simulink model "simulink_app"  (R2015a)
settings: Solver=FixedStepDiscrete  SolverMode=SingleTasking  StartTime=0.0  StopTime=inf  FixedStep=0.004  RelTol=1e-3
undefined symbols (not defined in the file): T_ctrl
libraries: simulink x6
settings Model: Creator=Adam  LastModifiedBy=David
settings SolverCC: AutoInsertRateTranBlk=on
settings DataIOCC: LimitDataPoints=off  SignalLoggingSaveFormat=ModelDataLogs  SaveOutput=off  SignalLogging=off  DSMLogging=off  SaveTime=off
settings OptimizationCC: InlineParams=on  OptimizeModelRefInitCode=on  LifeSpan=Inf
settings DebuggingCC: UnderspecifiedInitializationDetection=Classic  MergeDetectMultiDrivingBlocksExec=none  SolverPrmCheckMsg=warning  MultiTaskDSMMsg=warning  MultiTaskCondExecSysMsg=none  UnconnectedInputMsg=none  UnconnectedOutputMsg=none  UnconnectedLineMsg=none  StateNameClashWarn=warning  StrictBusMsg=None
settings HardwareCC: ProdLargestAtomicInteger=Long  ProdLargestAtomicFloat=Float  ProdEndianess=LittleEndian  ProdHWDeviceType=ARM Compatible->ARM 7
settings RTWCC: SystemTargetFile=ert.tlc  GenCodeOnly=on  GenerateMakefile=off  TemplateMakefile=ert_default_tmf  Description=Embedded Coder  RTWVerbose=off  RTWCompilerOptimization=on
settings RTWCC: CustomSourceCode=|
  | // Simulink wrapper code for PX4 (PX4FMU & Pixhawk)
  | // Developed by Adam Polak, Polakium Engineering 2014
  | // http://www.polakiumengineering.org
  | 
  | #include <nuttx/config.h>
  | #include <poll.h>
  | #include <stdio.h>
  | #include <stdlib.h>
  | #include <unistd.h>
  | #include <uORB/uORB.h>
  | #include <uORB/topics/sensor_combined.h>
  | #include <uORB/topics/vehicle_attitude.h>
  | #include <uORB/topics/optical_flow.h>
  | #include <uORB/topics/vehicle_gps_position.h>
  | #include <drivers/drv_led.h>
  | #include <drivers/drv_rgbled.h>
  | #include <drivers/drv_pwm_output.h>
  | #include <drivers/drv_rc_input.h>
  | #include <drivers/drv_hrt.h>
  | #include <systemlib/systemlib.h>
  | 
  | __EXPORT int simulink_app_main(int argc, char *argv[]);
  | 
  | const char *dev_rgbled = RGBLED_DEVICE_PATH;
  | const char *dev_pwm = PWM_OUTPUT_DEVICE_PATH;
  | 
  | static int simulink_task;
  | static bool thread_exit;
  | static bool pwm_enabled;
  | 
  | struct rgbled_rgbset_t{
  |   uint8_t red;
  |   uint8_t green;
  |   uint8_t blue;
  | };
  | 
  | int step_size = 4; // fundamental sample time (ms)
  | int i = 1;
  | 
  | int simulink_main(int argc, char *argv[])
  | {
  |   simulink_app_initialize();
  | 
  |   // declare data subscriptions
  |   int sensors_sub = orb_subscribe(ORB_ID(sensor_combined));
  |   int pwm_inputs_sub = orb_subscribe(ORB_ID(input_rc));
  |   int attitude_sub = orb_subscribe(ORB_ID(vehicle_attitude));
  |   int flow_sub = orb_subscribe(ORB_ID(optical_flow));
  |   int gps_sub = orb_subscribe(ORB_ID(vehicle_gps_position));
  | 
  |   struct sensor_combined_s sensors;
  |   struct rc_input_values pwm_inputs;
  |   struct vehicle_attitude_s attitude;
  |   struct optical_flow_s flow;
  |   struct vehicle_gps_position_s gps;
  | 
  |   orb_set_interval(sensors_sub, step_size);
  | 
  |   // declare output devices
  |   int rgbled = open(dev_rgbled, 0);
  |   int pwm = open(dev_pwm, 0);
  | 
  |   // initialize outputs
  |   ioctl(rgbled, RGBLED_SET_MODE, (unsigned long)RGBLED_MODE_ON);
  |   ioctl(pwm, PWM_SERVO_SET_ARM_OK, 0);
  |   ioctl(pwm, PWM_SERVO_ARM, 0);
  |   pwm_enabled = 0;
  | 
  |   struct pollfd fds[] = {
  |     { .fd = sensors_sub, .events = POLLIN },
  |   };
  | 
  |   // primary application thread
  |   while (!thread_exit) {
  |     int poll_return = poll(fds, 1, 1000);
  |     if (poll_return > 0) {
  |       if (fds[0].revents & POLLIN) {
  |         // assign sensor data
  |         orb_copy(ORB_ID(sensor_combined), sensors_sub, &sensors);
  |         orb_copy(ORB_ID(vehicle_attitude), attitude_sub, &attitude);
  |         orb_copy(ORB_ID(optical_flow), flow_sub, &flow);
  |         orb_copy(ORB_ID(vehicle_gps_position), gps_sub, &gps);
  |         orb_copy(ORB_ID(input_rc), pwm_inputs_sub, &pwm_inputs);
  |         simulink_app_U.runtime = hrt_absolute_time();
  |         simulink_app_U.mag_x = sensors.magnetometer_ga[0];
  |         simulink_app_U.mag_y = sensors.magnetometer_ga[1];
  |         simulink_app_U.mag_z = sensors.magnetometer_ga[2];
  |         simulink_app_U.acc_x = sensors.accelerometer_m_s2[0];
  |         simulink_app_U.acc_y = sensors.accelerometer_m_s2[1];
  |         simulink_app_U.acc_z = sensors.accelerometer_m_s2[2];
  |         simulink_app_U.gyro_x = sensors.gyro_rad_s[0];
  |         simulink_app_U.gyro_y = sensors.gyro_rad_s[1];
  |         simulink_app_U.gyro_z = sensors.gyro_rad_s[2];
  |         simulink_app_U.rate_roll = attitude.rollspeed;
  |         simulink_app_U.rate_pitch = attitude.pitchspeed;
  |         simulink_app_U.rate_yaw = attitude.yawspeed;
  |         simulink_app_U.att_roll = attitude.roll;
  |         simulink_app_U.att_pitch = attitude.pitch;
  |         simulink_app_U.att_yaw = attitude.yaw;
  |         simulink_app_U.q0 = attitude.q[0];
  |         simulink_app_U.q1 = attitude.q[1];
  |         simulink_app_U.q2 = attitude.q[2];
  |         simulink_app_U.q3 = attitude.q[3];
  |         simulink_app_U.baro_alt = sensors.baro_alt_meter;
  |         simulink_app_U.sonar_dist = flow.ground_distance_m;
  |         simulink_app_U.flow_x = flow.flow_comp_x_m;
  |         simulink_app_U.flow_y = flow.flow_comp_y_m;
  |         simulink_app_U.gps_sat = gps.satellites_used;
  |         simulink_app_U.gps_lat = 0.0000001*(double)gps.lat;
  |         simulink_app_U.gps_lon = 0.0000001*(double)gps.lon;
  |         simulink_app_U.gps_alt = 0.001*(double)gps.alt;
  |         simulink_app_U.gps_vel = gps.vel_m_s;
  |         simulink_app_U.gps_vel_n = gps.vel_n_m_s;
  |         simulink_app_U.gps_vel_e = gps.vel_e_m_s;
  |         simulink_app_U.gps_vel_d = gps.vel_d_m_s;
  |         simulink_app_U.ch1 = pwm_inputs.values[0];
  |         simulink_app_U.ch2 = pwm_inputs.values[1];
  |         simulink_app_U.ch3 = pwm_inputs.values[2];
  |         simulink_app_U.ch4 = pwm_inputs.values[3];
  |         simulink_app_U.ch5 = pwm_inputs.values[4];
  |         simulink_app_U.ch6 = pwm_inputs.values[5];
  |         simulink_app_U.ch7 = pwm_inputs.values[6];
  |         simulink_app_U.ch8 = pwm_inputs.values[7];
  |         if (i < 25) { // 10Hz loop
  |           i = i++;
  |         } else {
  |           // check arm state
  |           if (simulink_app_Y.pwm_arm == 1 && pwm_enabled == 0) {
  |             // arm system
  |             pwm_enabled = 1;
  |             printf("\t  ARMED\t\t  ARMED\t\t  ARMED\t\t  ARMED\t\t  ARMED\t\t  ARMED\t\t  ARMED\t\t  ARMED\n");
  |           } else if (simulink_app_Y.pwm_arm == 0 && pwm_enabled == 1) {
  |             // disarm system
  |             ioctl(pwm, PWM_SERVO_SET(0), 1000);
  |             ioctl(pwm, PWM_SERVO_SET(1), 1000);
  |             ioctl(pwm, PWM_SERVO_SET(2), 1000);
  |             ioctl(pwm, PWM_SERVO_SET(3), 1000);
  |             ioctl(pwm, PWM_SERVO_SET(4), 1000);
  |             ioctl(pwm, PWM_SERVO_SET(5), 1000);
  |             ioctl(pwm, PWM_SERVO_SET(6), 1000);
  |             ioctl(pwm, PWM_SERVO_SET(7), 1000);
  |             pwm_enabled = 0;
  |             printf("\tDISARMED\tDISARMED\tDISARMED\tDISARMED\tDISARMED\tDISARMED\tDISARMED\tDISARMED\n");
  |           }
  |           // output FMU LED signals
  |           if (simulink_app_Y.led_blue == 1) {
  |             led_on(LED_BLUE);
  |           } else {
  |             led_off(LED_BLUE);
  |           }
  |           if (simulink_app_Y.led_red == 1) {
  |             led_on(LED_RED);
  |           } else {
  |             led_off(LED_RED);
  |           }
  |           // output RGBLED signals
  |           rgbled_rgbset_t rgb_value;
  |           rgb_value.red = simulink_app_Y.rgb_red;
  |           rgb_value.green = simulink_app_Y.rgb_green;
  |           rgb_value.blue = simulink_app_Y.rgb_blue;
  |           ioctl(rgbled, RGBLED_SET_RGB, (unsigned long)&rgb_value);
  |           //print debug data
  |           printf("%8.4f\t%8.4f\t%8.4f\t%8.4f\t%8.4f\t%8.4f\t%8.4f\t%8.4f\t%8.4f\n",
  |               (double)(simulink_app_U.runtime/1000000),
  |               (double)simulink_app_Y.debug1,
  |               (double)simulink_app_Y.debug2,
  |               (double)simulink_app_Y.debug3,
  |               (double)simulink_app_Y.debug4,
  |               (double)simulink_app_Y.debug5,
  |               (double)simulink_app_Y.debug6,
  |               (double)simulink_app_Y.debug7,
  |               (double)simulink_app_Y.debug8);
  |           i = 1;
  |         }
  |         // output pwm signals
  |         if (pwm_enabled == 1) {
  |           ioctl(pwm, PWM_SERVO_SET(0), simulink_app_Y.pwm1);
  |           ioctl(pwm, PWM_SERVO_SET(1), simulink_app_Y.pwm2);
  |           ioctl(pwm, PWM_SERVO_SET(2), simulink_app_Y.pwm3);
  |           ioctl(pwm, PWM_SERVO_SET(3), simulink_app_Y.pwm4);
  |           ioctl(pwm, PWM_SERVO_SET(4), simulink_app_Y.pwm5);
  |           ioctl(pwm, PWM_SERVO_SET(5), simulink_app_Y.pwm6);
  |           ioctl(pwm, PWM_SERVO_SET(6), simulink_app_Y.pwm7);
  |           ioctl(pwm, PWM_SERVO_SET(7), simulink_app_Y.pwm8);
  |         } else {
  |           ioctl(pwm, PWM_SERVO_SET(0), 1000);
  |           ioctl(pwm, PWM_SERVO_SET(1), 1000);
  |           ioctl(pwm, PWM_SERVO_SET(2), 1000);
  |           ioctl(pwm, PWM_SERVO_SET(3), 1000);
  |           ioctl(pwm, PWM_SERVO_SET(4), 1000);
  |           ioctl(pwm, PWM_SERVO_SET(5), 1000);
  |           ioctl(pwm, PWM_SERVO_SET(6), 1000);
  |           ioctl(pwm, PWM_SERVO_SET(7), 1000);
  |         }
  |         // execute simulink code
  |         simulink_app_step();
  |       }
  |     }
  |   }
  |   // disable pwm outputs
  |   ioctl(pwm, PWM_SERVO_SET(0), 1000);
  |   ioctl(pwm, PWM_SERVO_SET(1), 1000);
  |   ioctl(pwm, PWM_SERVO_SET(2), 1000);
  |   ioctl(pwm, PWM_SERVO_SET(3), 1000);
  |   ioctl(pwm, PWM_SERVO_SET(4), 1000);
  |   ioctl(pwm, PWM_SERVO_SET(5), 1000);
  |   ioctl(pwm, PWM_SERVO_SET(6), 1000);
  |   ioctl(pwm, PWM_SERVO_SET(7), 1000);
  |   ioctl(pwm, PWM_SERVO_DISARM, 0);
  |   // disable LEDs
  |   led_off(LED_BLUE);
  |   led_off(LED_RED);
  |   ioctl(rgbled, RGBLED_SET_MODE, (unsigned long)RGBLED_MODE_OFF);
  |   // close sensor subscriptions
  |   close(sensors_sub);
  |   close(attitude_sub);
  |   close(flow_sub);
  |   close(pwm_inputs_sub);
  |   close(gps_sub);
  |   // terminate application thread
  |   exit(0);
  | }
  | 
  | int simulink_app_main(int argc, char *argv[])
  | {
  |   // start primary application thread
  |   if (!strcmp(argv[1], "start")) {
  |     thread_exit = false;
  |     simulink_task = task_spawn_cmd("simulink_app",
  |       SCHED_DEFAULT,
  |       SCHED_PRIORITY_MAX - 15,
  |       10240,
  |       simulink_main,
  |       NULL);
  |     exit(0);
  |   }
  | 
  |   // terminate primary application thread
  |   if (!strcmp(argv[1], "stop")) {
  |     thread_exit = true;
  |     exit(0);
  |   }
  | 
  |   exit(1);
  | }
settings CodeAppCC: IgnoreCustomStorageClasses=off  SimulinkBlockComments=off
settings ERTTargetCC: GenerateSampleERTMain=off  ParMdlRefBuildCompliant=on  CompOptLevelCompliant=on  ConcurrentExecutionCompliant=on  ERTFirstTimeCompliant=on  SupportContinuousTime=off  SupportVariableSizeSignals=off  ParenthesesLevel=Minimum  ModelStepFunctionPrototypeControlCompliant=on  CPPClassGenCompliant=on  InlinedParameterPlacement=Hierarchical  ERTCustomFileTemplate=example_file_process.tlc  GlobalDataDefinition=InSourceFile  GlobalDataReference=InSourceFile  ERTFilePackagingFormat=Compact  PreserveExternInFcnDecls=off

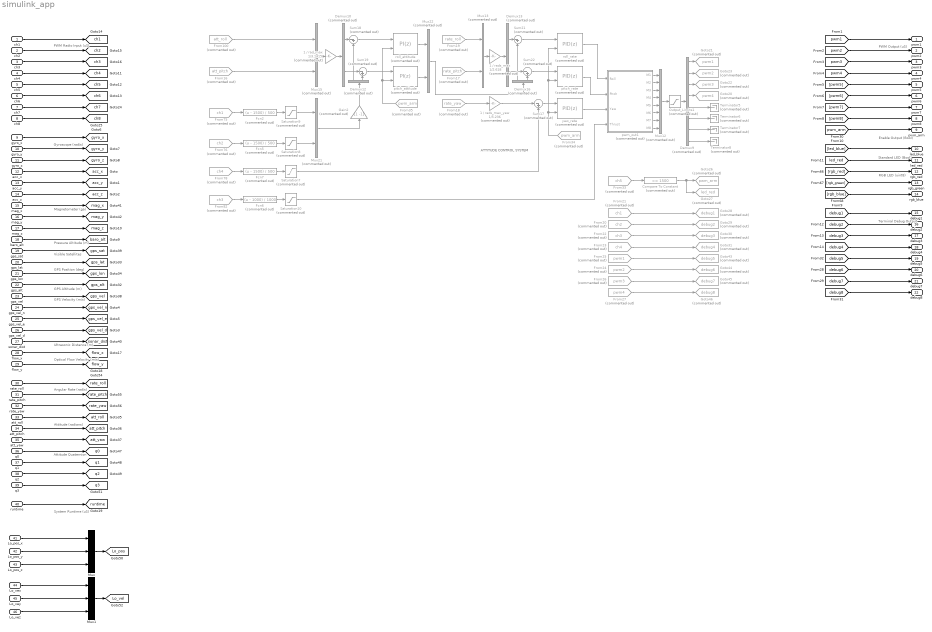
== system simulink_app ==
  note: Terminal Debug Output
  note: RGB LED (uint8)
  note: Standard LED (Bool)
  note: PWM Output (uS)
  note: Enable Output (Bool)
  note: GPS Velocity (m/s)
  note: GPS Altitude (m)
  note: GPS Position (deg)
  note: Attitude Quaternion
  note: Attitude (radians)
  note: Angular Rate (rad/s)
  note: Optical Flow Velocity (m/s)
  note: Ultrasonic Distance (m)
  note: Pressure Altitude (m)
  note: Magnetometer (ga)
  note: System Runtime (uS)
  note: Gyroscope (rad/s)
  note: PWM Radio Input (uS)
  note: Visible Satellites
  note: ATTITUDE CONTROL SYSTEM
  ch1 : Inport
  ch2 : Inport  Port=2
  ch3 : Inport  Port=3
  ch4 : Inport  Port=4
  ch5 : Inport  Port=5
  ch6 : Inport  Port=6
  ch7 : Inport  Port=7
  ch8 : Inport  Port=8
  gyro_x : Inport  Port=9
  gyro_y : Inport  Port=10
  gyro_z : Inport  Port=11
  acc_x : Inport  Port=12
  acc_y : Inport  Port=13
  acc_z : Inport  Port=14
  mag_x : Inport  Port=15
  mag_y : Inport  Port=16
  mag_z : Inport  Port=17
  baro_alt : Inport  Port=18
  gps_sat : Inport  Port=19
  gps_lat : Inport  Port=20
  gps_lon : Inport  Port=21
  gps_alt : Inport  Port=22
  gps_vel : Inport  Port=23
  gps_vel_n : Inport  Port=24
  gps_vel_e : Inport  Port=25
  gps_vel_d : Inport  Port=26
  sonar_dist : Inport  Port=27
  flow_x : Inport  Port=28
  flow_y : Inport  Port=29
  rate_roll : Inport  Port=30
  rate_pitch : Inport  Port=31
  rate_yaw : Inport  Port=32
  att_roll : Inport  Port=33
  att_pitch : Inport  Port=34
  att_yaw : Inport  Port=35
  q0 : Inport  Port=36
  q1 : Inport  Port=37
  q2 : Inport  Port=38
  q3 : Inport  Port=39
  runtime : Inport  Port=40
  Lo_pos_x : Inport  Port=41  PortDimensions=[1,1]  SampleTime=T_ctrl
  Lo_pos_y : Inport  Port=42  PortDimensions=[1,1]  SampleTime=T_ctrl
  Lo_pos_z : Inport  Port=43  PortDimensions=[1,1]  SampleTime=T_ctrl
  Lo_vex : Inport  Port=44  PortDimensions=[1,1]  SampleTime=T_ctrl
  Lo_vey : Inport  Port=45  PortDimensions=[1,1]  SampleTime=T_ctrl
  Lo_vez : Inport  Port=46  PortDimensions=[1,1]  SampleTime=T_ctrl
  1 / rad_max : Gain  Commented=on  Gain=1/3.1415
  1 / rads_max : Gain  Commented=on  Gain=1/2.618
  1 / rads_max_yaw : Gain  Commented=on  Gain=1/5.236
  Compare To Constant : simulink/Logic and Bit Operations/Compare To Constant  Commented=on  relop=>=  const=1500  OutDataTypeStr=boolean
  Demux{10,12..13,16} (4 alike) : Demux  Commented=on  Outputs=2
  Demux9 : Demux  Commented=on  Outputs=8
  Fcn2 : Fcn  Commented=on  Expr=(u - 1500) / 500
  Fcn5 : Fcn  Commented=on  Expr=(u - 1500) / 500
  Fcn6 : Fcn  Commented=on  Expr=(u - 1000) / 1000
  Fcn7 : Fcn  Commented=on  Expr=(u - 1500) / 500
  From100 : From  Commented=on  GotoTag=att_roll  TagVisibility=global
  From16 : From  Commented=on  GotoTag=att_pitch  TagVisibility=global
  From17 : From  Commented=on  GotoTag=rate_pitch  TagVisibility=global
  From18 : From  Commented=on  GotoTag=rate_yaw  TagVisibility=global
  From19 : From  Commented=on  GotoTag=rate_roll  TagVisibility=global
  From20 : From  Commented=on  GotoTag=ch2  TagVisibility=global
  From21 : From  Commented=on  GotoTag=ch1  TagVisibility=global
  From22 : From  Commented=on  GotoTag=ch3  TagVisibility=global
  From23 : From  Commented=on  GotoTag=ch4  TagVisibility=global
  From24 : From  Commented=on  GotoTag=pwm2  TagVisibility=global
  From25 : From  Commented=on  GotoTag=pwm1  TagVisibility=global
  From26 : From  Commented=on  GotoTag=pwm3  TagVisibility=global
  From27 : From  Commented=on  GotoTag=pwm4  TagVisibility=global
  From33 : From  Commented=on  GotoTag=ch5  TagVisibility=global
  From34 : From  Commented=on  GotoTag=pwm_arm  TagVisibility=global
  From35 : From  Commented=on  GotoTag=pwm_arm  TagVisibility=global
  From75 : From  Commented=on  GotoTag=ch1  TagVisibility=global
  From76 : From  Commented=on  GotoTag=ch2  TagVisibility=global
  From78 : From  Commented=on  GotoTag=ch4  TagVisibility=global
  From82 : From  Commented=on  GotoTag=ch3  TagVisibility=global
  Gain2 : Gain  Commented=on  Gain=[1 -1]
  Goto20 : Goto  Commented=on  GotoTag=pwm4  TagVisibility=global
  Goto21 : Goto  Commented=on  GotoTag=pwm1  TagVisibility=global
  Goto22 : Goto  Commented=on  GotoTag=pwm3  TagVisibility=global
  Goto23 : Goto  Commented=on  GotoTag=pwm2  TagVisibility=global
  Goto26 : Goto  Commented=on  GotoTag=pwm_arm  TagVisibility=global
  Goto27 : Goto  Commented=on  GotoTag=led_red  TagVisibility=global
  Goto28 : Goto  Commented=on  GotoTag=debug1  TagVisibility=global
  Goto29 : Goto  Commented=on  GotoTag=debug2  TagVisibility=global
  Goto30 : Goto  Commented=on  GotoTag=debug3  TagVisibility=global
  Goto31 : Goto  Commented=on  GotoTag=debug4  TagVisibility=global
  Goto43 : Goto  Commented=on  GotoTag=debug5  TagVisibility=global
  Goto44 : Goto  Commented=on  GotoTag=debug6  TagVisibility=global
  Goto45 : Goto  Commented=on  GotoTag=debug7  TagVisibility=global
  Goto46 : Goto  Commented=on  GotoTag=debug8  TagVisibility=global
  Mux : Mux  Inputs=3
  Mux1 : Mux  Inputs=3
  Mux12 : Mux  Commented=on  Inputs=8
  Mux{13,15,21..22} (4 alike) : Mux  Commented=on  Inputs=2
  Output_Limits1 : Saturate  Commented=on  UpperLimit=2000  LowerLimit=1000
  Saturation10 : Saturate  Commented=on  UpperLimit=1  LowerLimit=0
  Saturation7 : Saturate  Commented=on  UpperLimit=1  LowerLimit=-1
  Saturation8 : Saturate  Commented=on  UpperLimit=1  LowerLimit=-1
  Saturation9 : Saturate  Commented=on  UpperLimit=1  LowerLimit=-1
  Sum{17..19,21..22} (5 alike) : Sum  Commented=on  Inputs=|-+
  Terminator{5..8} (4 alike) : Terminator  Commented=on
  pitch_attitude : simulink/Continuous/PID Controller  Commented=on  Controller=PI  TimeDomain=Discrete-time  SampleTime=-1  IntegratorMethod=Forward Euler  FilterMethod=Forward Euler  Form=Parallel  UseFilter=on  ControllerParametersSource=internal  P=0.70  I=0  D=0  N=100  InitialConditionSource=internal  InitialConditionForIntegrator=0  InitialConditionForFilter=0  ExternalReset=either  LimitOutput=on  UpperSaturationLimit=1  LowerSaturationLimit=-1  LinearizeAsGain=on  AntiWindupMode=none  Kb=1  TrackingMode=off  Kt=1  PParamMin=[]  PParamMax=[]  IParamMin=[]  IParamMax=[]  DParamMin=[]  DParamMax=[]  NParamMin=[]  NParamMax=[]  KbParamMin=[]  KbParamMax=[]  KtParamMin=[]  KtParamMax=[]  POutMin=[]  POutMax=[]  IOutMin=[]  IOutMax=[]  DOutMin=[]  DOutMax=[]  NOutMin=[]  NOutMax=[]  KbOutMin=[]  KbOutMax=[]  KtOutMin=[]  KtOutMax=[]  IntegratorOutMin=[]  IntegratorOutMax=[]  FilterOutMin=[]  FilterOutMax=[]  SumOutMin=[]  SumOutMax=[]  SumI1OutMin=[]  SumI1OutMax=[]  SumI2OutMin=[]  SumI2OutMax=[]  SumI3OutMin=[]  SumI3OutMax=[]  SumDOutMin=[]  SumDOutMax=[]  SaturationOutMin=[]  SaturationOutMax=[]  IntegratorContinuousStateAttributes=''  IntegratorStateMustResolveToSignalObject=off  IntegratorRTWStateStorageClass=Auto  FilterContinuousStateAttributes=''  FilterStateMustResolveToSignalObject=off  FilterRTWStateStorageClass=Auto  DifferentiatorICPrevScaledInput=0  DifferentiatorOutMin=[]  DifferentiatorOutMax=[]
  pitch_rate : simulink/Continuous/PID Controller  Commented=on  Controller=PID  TimeDomain=Discrete-time  SampleTime=-1  IntegratorMethod=Forward Euler  FilterMethod=Forward Euler  Form=Parallel  UseFilter=on  ControllerParametersSource=internal  P=0.45  I=0.45  D=0.003  N=100  InitialConditionSource=internal  InitialConditionForIntegrator=0  InitialConditionForFilter=0  ExternalReset=either  LimitOutput=on  UpperSaturationLimit=1  LowerSaturationLimit=-1  LinearizeAsGain=on  AntiWindupMode=none  Kb=1  TrackingMode=off  Kt=1  PParamMin=[]  PParamMax=[]  IParamMin=[]  IParamMax=[]  DParamMin=[]  DParamMax=[]  NParamMin=[]  NParamMax=[]  KbParamMin=[]  KbParamMax=[]  KtParamMin=[]  KtParamMax=[]  POutMin=[]  POutMax=[]  IOutMin=[]  IOutMax=[]  DOutMin=[]  DOutMax=[]  NOutMin=[]  NOutMax=[]  KbOutMin=[]  KbOutMax=[]  KtOutMin=[]  KtOutMax=[]  IntegratorOutMin=[]  IntegratorOutMax=[]  FilterOutMin=[]  FilterOutMax=[]  SumOutMin=[]  SumOutMax=[]  SumI1OutMin=[]  SumI1OutMax=[]  SumI2OutMin=[]  SumI2OutMax=[]  SumI3OutMin=[]  SumI3OutMax=[]  SumDOutMin=[]  SumDOutMax=[]  SaturationOutMin=[]  SaturationOutMax=[]  IntegratorContinuousStateAttributes=''  IntegratorStateMustResolveToSignalObject=off  IntegratorRTWStateStorageClass=Auto  FilterContinuousStateAttributes=''  FilterStateMustResolveToSignalObject=off  FilterRTWStateStorageClass=Auto  DifferentiatorICPrevScaledInput=0  DifferentiatorOutMin=[]  DifferentiatorOutMax=[]
  pwm_out1 : MATLAB Function  Commented=on  TreatAsAtomicUnit=on  SystemSampleTime=0.004
  roll_attitude : simulink/Continuous/PID Controller  Commented=on  Controller=PI  TimeDomain=Discrete-time  SampleTime=-1  IntegratorMethod=Forward Euler  FilterMethod=Forward Euler  Form=Parallel  UseFilter=on  ControllerParametersSource=internal  P=0.70  I=0  D=0  N=100  InitialConditionSource=internal  InitialConditionForIntegrator=0  InitialConditionForFilter=0  ExternalReset=either  LimitOutput=on  UpperSaturationLimit=1  LowerSaturationLimit=-1  LinearizeAsGain=on  AntiWindupMode=none  Kb=1  TrackingMode=off  Kt=1  PParamMin=[]  PParamMax=[]  IParamMin=[]  IParamMax=[]  DParamMin=[]  DParamMax=[]  NParamMin=[]  NParamMax=[]  KbParamMin=[]  KbParamMax=[]  KtParamMin=[]  KtParamMax=[]  POutMin=[]  POutMax=[]  IOutMin=[]  IOutMax=[]  DOutMin=[]  DOutMax=[]  NOutMin=[]  NOutMax=[]  KbOutMin=[]  KbOutMax=[]  KtOutMin=[]  KtOutMax=[]  IntegratorOutMin=[]  IntegratorOutMax=[]  FilterOutMin=[]  FilterOutMax=[]  SumOutMin=[]  SumOutMax=[]  SumI1OutMin=[]  SumI1OutMax=[]  SumI2OutMin=[]  SumI2OutMax=[]  SumI3OutMin=[]  SumI3OutMax=[]  SumDOutMin=[]  SumDOutMax=[]  SaturationOutMin=[]  SaturationOutMax=[]  IntegratorContinuousStateAttributes=''  IntegratorStateMustResolveToSignalObject=off  IntegratorRTWStateStorageClass=Auto  FilterContinuousStateAttributes=''  FilterStateMustResolveToSignalObject=off  FilterRTWStateStorageClass=Auto  DifferentiatorICPrevScaledInput=0  DifferentiatorOutMin=[]  DifferentiatorOutMax=[]
  roll_rate : simulink/Continuous/PID Controller  Commented=on  Controller=PID  TimeDomain=Discrete-time  SampleTime=-1  IntegratorMethod=Forward Euler  FilterMethod=Forward Euler  Form=Parallel  UseFilter=on  ControllerParametersSource=internal  P=0.45  I=0.45  D=0.003  N=100  InitialConditionSource=internal  InitialConditionForIntegrator=0  InitialConditionForFilter=0  ExternalReset=either  LimitOutput=on  UpperSaturationLimit=1  LowerSaturationLimit=-1  LinearizeAsGain=on  AntiWindupMode=none  Kb=1  TrackingMode=off  Kt=1  PParamMin=[]  PParamMax=[]  IParamMin=[]  IParamMax=[]  DParamMin=[]  DParamMax=[]  NParamMin=[]  NParamMax=[]  KbParamMin=[]  KbParamMax=[]  KtParamMin=[]  KtParamMax=[]  POutMin=[]  POutMax=[]  IOutMin=[]  IOutMax=[]  DOutMin=[]  DOutMax=[]  NOutMin=[]  NOutMax=[]  KbOutMin=[]  KbOutMax=[]  KtOutMin=[]  KtOutMax=[]  IntegratorOutMin=[]  IntegratorOutMax=[]  FilterOutMin=[]  FilterOutMax=[]  SumOutMin=[]  SumOutMax=[]  SumI1OutMin=[]  SumI1OutMax=[]  SumI2OutMin=[]  SumI2OutMax=[]  SumI3OutMin=[]  SumI3OutMax=[]  SumDOutMin=[]  SumDOutMax=[]  SaturationOutMin=[]  SaturationOutMax=[]  IntegratorContinuousStateAttributes=''  IntegratorStateMustResolveToSignalObject=off  IntegratorRTWStateStorageClass=Auto  FilterContinuousStateAttributes=''  FilterStateMustResolveToSignalObject=off  FilterRTWStateStorageClass=Auto  DifferentiatorICPrevScaledInput=0  DifferentiatorOutMin=[]  DifferentiatorOutMax=[]
  yaw_rate : simulink/Continuous/PID Controller  Commented=on  Controller=PID  TimeDomain=Discrete-time  SampleTime=-1  IntegratorMethod=Forward Euler  FilterMethod=Forward Euler  Form=Parallel  UseFilter=on  ControllerParametersSource=internal  P=1.05  I=1.05  D=0  N=100  InitialConditionSource=internal  InitialConditionForIntegrator=0  InitialConditionForFilter=0  ExternalReset=either  LimitOutput=on  UpperSaturationLimit=1  LowerSaturationLimit=-1  LinearizeAsGain=on  AntiWindupMode=none  Kb=1  TrackingMode=off  Kt=1  PParamMin=[]  PParamMax=[]  IParamMin=[]  IParamMax=[]  DParamMin=[]  DParamMax=[]  NParamMin=[]  NParamMax=[]  KbParamMin=[]  KbParamMax=[]  KtParamMin=[]  KtParamMax=[]  POutMin=[]  POutMax=[]  IOutMin=[]  IOutMax=[]  DOutMin=[]  DOutMax=[]  NOutMin=[]  NOutMax=[]  KbOutMin=[]  KbOutMax=[]  KtOutMin=[]  KtOutMax=[]  IntegratorOutMin=[]  IntegratorOutMax=[]  FilterOutMin=[]  FilterOutMax=[]  SumOutMin=[]  SumOutMax=[]  SumI1OutMin=[]  SumI1OutMax=[]  SumI2OutMin=[]  SumI2OutMax=[]  SumI3OutMin=[]  SumI3OutMax=[]  SumDOutMin=[]  SumDOutMax=[]  SaturationOutMin=[]  SaturationOutMax=[]  IntegratorContinuousStateAttributes=''  IntegratorStateMustResolveToSignalObject=off  IntegratorRTWStateStorageClass=Auto  FilterContinuousStateAttributes=''  FilterStateMustResolveToSignalObject=off  FilterRTWStateStorageClass=Auto  DifferentiatorICPrevScaledInput=0  DifferentiatorOutMin=[]  DifferentiatorOutMax=[]
  pwm1 : Outport
  pwm2 : Outport  Port=2
  pwm3 : Outport  Port=3
  pwm4 : Outport  Port=4
  pwm5 : Outport  Port=5
  pwm6 : Outport  Port=6
  pwm7 : Outport  Port=7
  pwm8 : Outport  Port=8
  pwm_arm : Outport  Port=9
  led_blue : Outport  Port=10  OutDataTypeStr=boolean
  led_red : Outport  Port=11  OutDataTypeStr=boolean
  rgb_red : Outport  Port=12  OutDataTypeStr=uint8
  rgb_green : Outport  Port=13  OutDataTypeStr=uint8
  rgb_blue : Outport  Port=14  OutDataTypeStr=uint8
  debug1 : Outport  Port=15
  debug2 : Outport  Port=16
  debug3 : Outport  Port=17
  debug4 : Outport  Port=18
  debug5 : Outport  Port=19
  debug6 : Outport  Port=20
  debug7 : Outport  Port=21
  debug8 : Outport  Port=22
  tag scope: Lo_pos=global, Lo_vel=global, acc_x=global, acc_y=global, acc_z=global, att_pitch=global, att_roll=global, att_yaw=global, baro_alt=global, ch1=global, ch2=global, ch3=global, ch4=global, ch5=global, ch6=global, ch7=global, ch8=global, flow_x=global, flow_y=global, gps_alt=global, gps_lat=global, gps_lon=global, gps_sat=global, gps_vel=global, gps_vel_d=global, gps_vel_e=global, gps_vel_n=global, gyro_x=global, gyro_y=global, gyro_z=global, mag_x=global, mag_y=global, mag_z=global, q0=global, q1=global, q2=global, q3=global, rate_pitch=global, rate_roll=global, rate_yaw=global, runtime=global, sonar_dist=global
  wires:
  [pwm1] -> pwm1/1
  [pwm2] -> pwm2/1
  [pwm3] -> pwm3/1
  [pwm4] -> pwm4/1
  [pwm5] -> pwm5/1
  [pwm6] -> pwm6/1
  [pwm7] -> pwm7/1
  [pwm8] -> pwm8/1
  [led_blue] -> led_blue/1
  [led_red] -> led_red/1
  [debug1] -> debug1/1
  [debug2] -> debug2/1
  [debug3] -> debug3/1
  [debug4] -> debug4/1
  [pwm_arm] -> pwm_arm/1
  [rgb_red] -> rgb_red/1
  [rgb_green] -> rgb_green/1
  [rgb_blue] -> rgb_blue/1
  sonar_dist/1 -> [sonar_dist]
  baro_alt/1 -> [baro_alt]
  gyro_z/1 -> [gyro_z]
  gyro_y/1 -> [gyro_y]
  gyro_x/1 -> [gyro_x]
  acc_z/1 -> [acc_z]
  acc_y/1 -> [acc_y]
  acc_x/1 -> [acc_x]
  mag_x/1 -> [mag_x]
  mag_y/1 -> [mag_y]
  mag_z/1 -> [mag_z]
  ch1/1 -> [ch1]
  ch2/1 -> [ch2]
  ch3/1 -> [ch3]
  ch4/1 -> [ch4]
  ch5/1 -> [ch5]
  ch6/1 -> [ch6]
  flow_y/1 -> [flow_y]
  flow_x/1 -> [flow_x]
  runtime/1 -> [runtime]
  ch7/1 -> [ch7]
  ch8/1 -> [ch8]
  att_roll/1 -> [att_roll]
  att_pitch/1 -> [att_pitch]
  att_yaw/1 -> [att_yaw]
  q0/1 -> [q0]
  q1/1 -> [q1]
  q2/1 -> [q2]
  q3/1 -> [q3]
  rate_roll/1 -> [rate_roll]
  rate_pitch/1 -> [rate_pitch]
  rate_yaw/1 -> [rate_yaw]
  gps_vel_n/1 -> [gps_vel_n]
  gps_vel_e/1 -> [gps_vel_e]
  gps_vel_d/1 -> [gps_vel_d]
  gps_lat/1 -> [gps_lat]
  gps_lon/1 -> [gps_lon]
  gps_alt/1 -> [gps_alt]
  gps_vel/1 -> [gps_vel]
  gps_sat/1 -> [gps_sat]
  [debug6] -> debug6/1
  [debug7] -> debug7/1
  [debug8] -> debug8/1
  [debug5] -> debug5/1
  From21/1 -> Goto28/1
  From20/1 -> Goto29/1
  From22/1 -> Goto30/1
  From23/1 -> Goto31/1
  From25/1 -> Goto43/1
  From24/1 -> Goto44/1
  From26/1 -> Goto45/1
  From27/1 -> Goto46/1
  pwm_out1/8(M8) -> Mux12/8
  pwm_out1/7(M7) -> Mux12/7
  pwm_out1/6(M6) -> Mux12/6
  pwm_out1/5(M5) -> Mux12/5
  pwm_out1/4(M4) -> Mux12/4
  pwm_out1/3(M3) -> Mux12/3
  pwm_out1/2(M2) -> Mux12/2
  pwm_out1/1(M1) -> Mux12/1
  Sum21/1 -> roll_rate/1
  1 / rads_max/1 -> Demux13/1
  Demux13/2 -> Sum22/1
  Demux13/1 -> Sum21/1
  Sum17/1 -> yaw_rate/1
  Sum22/1 -> pitch_rate/1
  Mux13/1 -> 1 / rads_max/1
  pitch_rate/1 -> pwm_out1/2(Pitch)
  Sum18/1 -> roll_attitude/1
  1 / rad_max/1 -> Demux10/1
  Demux10/2 -> Sum19/1
  Demux10/1 -> Sum18/1
  Mux12/1 -> Output_Limits1/1
  From19/1 -> Mux13/1
  Demux12/2 -> Sum19/2
  Demux12/1 -> Sum18/2
  Demux16/2 -> Sum22/2
  Demux16/1 -> Sum21/2
  roll_attitude/1 -> Mux22/1
  pitch_attitude/1 -> Mux22/2
  From18/1 -> 1 / rads_max_yaw/1
  From17/1 -> Mux13/2
  From75/1 -> Fcn2/1
  From76/1 -> Fcn5/1
  From78/1 -> Fcn7/1
  Fcn7/1 -> Saturation7/1
  Saturation9/1 -> Mux21/1
  Fcn5/1 -> Saturation8/1
  Fcn2/1 -> Saturation9/1
  Sum19/1 -> pitch_attitude/1
  Demux9/5 -> Terminator5/1
  Demux9/6 -> Terminator6/1
  Demux9/7 -> Terminator7/1
  Demux9/8 -> Terminator8/1
  roll_rate/1 -> pwm_out1/1(Roll)
  Demux9/1 -> Goto21/1
  Demux9/2 -> Goto23/1
  Demux9/3 -> Goto22/1
  Demux9/4 -> Goto20/1
  1 / rads_max_yaw/1 -> Sum17/1
  From82/1 -> Fcn6/1
  Fcn6/1 -> Saturation10/1
  Saturation8/1 -> Mux21/2
  Mux21/1 -> Gain2/1
  From16/1 -> Mux15/2
  Mux15/1 -> 1 / rad_max/1
  From100/1 -> Mux15/1
  yaw_rate/1 -> pwm_out1/3(Yaw)
  Gain2/1 -> Demux12/1
  Saturation7/1 -> Sum17/2
  Output_Limits1/1 -> Demux9/1
  From33/1 -> Compare To Constant/1
  Compare To Constant/1 -> Goto27/1, Goto26/1
  From34/1 -> pitch_rate/2, roll_rate/2, yaw_rate/2
  From35/1 -> pitch_attitude/2, roll_attitude/2
  Saturation10/1 -> pwm_out1/4(Thrust)
  Mux22/1 -> Demux16/1
  Lo_pos_x/1 -> Mux/1
  Lo_pos_y/1 -> Mux/2
  Lo_pos_z/1 -> Mux/3
  Lo_vex/1 -> Mux1/1
  Lo_vey/1 -> Mux1/2
  Lo_vez/1 -> Mux1/3
  Mux/1 -> [Lo_pos]
  Mux1/1 -> [Lo_vel]

== matlab function simulink_app/pwm_out1 ==
  data: Roll input; M1 output; Pitch input; Yaw input; Thrust input; M2 output; M3 output; M4 output; M5 output; M6 output; M7 output; M8 output
function [M1, M2, M3, M4, M5, M6, M7, M8] = motor_mixer(Roll, Pitch, Yaw, Thrust)

idle_PWM = 1000;

% Quad X
M1 = ((Roll + Pitch - Yaw) / 2 * Thrust + Thrust) * 1000 + idle_PWM;
M2 = ((-Roll + Pitch + Yaw) / 2 * Thrust + Thrust) * 1000 + idle_PWM;
M3 = ((-Roll - Pitch - Yaw) / 2 * Thrust + Thrust) * 1000 + idle_PWM;
M4 = ((Roll - Pitch + Yaw) / 2 * Thrust + Thrust) * 1000 + idle_PWM;
M5 = 1000;
M6 = 1000;
M7 = 1000;
M8 = 1000;

% Quad +
% M1 = ((Pitch - Yaw) * Thrust / 2 + Thrust) * 1000 + idle_PWM;
% M2 = ((-Roll + Yaw) * Thrust / 2 + Thrust) * 1000 + idle_PWM;
% M3 = ((-Pitch - Yaw) * Thrust / 2 + Thrust) * 1000 + idle_PWM;
% M4 = ((Roll + Yaw) * Thrust / 2 + Thrust) * 1000 + idle_PWM;
% M5 = 1000;
% M6 = 1000;
% M7 = 1000;
% M8 = 1000;

% Hex X
% M1 = ((Pitch + Roll / 2 - Yaw) * Thrust / 2 + Thrust) * 1000 + idle_PWM;
% M2 = ((Pitch - Roll / 2 + Yaw) * Thrust / 2 + Thrust) * 1000 + idle_PWM;
% M3 = ((-Roll - Yaw) * Thrust / 2 + Thrust) * 1000 + idle_PWM;
% M4 = ((-Pitch - Roll / 2 + Yaw) * Thrust / 2 + Thrust) * 1000 + idle_PWM;
% M5 = ((-Pitch + Roll / 2 - Yaw) * Thrust / 2 + Thrust) * 1000 + idle_PWM;
% M6 = ((Roll + Yaw) * Thrust / 2 + Thrust) * 1000 + idle_PWM;
% M7 = 1000;
% M8 = 1000;
